simulink model "ID"  (R2024b)
settings: Solver=FixedStepDiscrete  StartTime=0.0  StopTime=Inf  FixedStep=0.001  RelTol=1e-3
model workspace (MAT data in the model file):
  robot : robotics.RigidBodyTree (value not decoded)
libraries: robotmaniplib x3
settings Model: Creator=sung  LastModifiedBy=sung
settings HardwareCC: ProdBitPerLong=64  ProdHWDeviceType=Intel->x86-64 (Linux 64)
settings RTWCC: GenCodeOnly=on  Toolchain=CMake

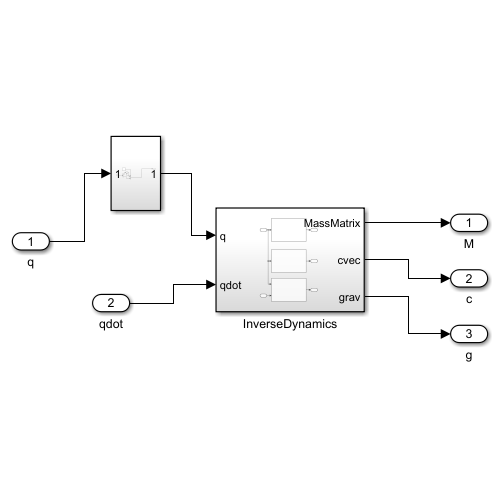
[thumbnail: Simulink's stored preview of the top-level diagram]
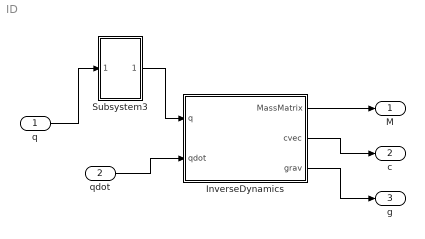
== system ID ==
  q : Inport
  qdot : Inport  Port=2
  InverseDynamics : Subsystem
  Subsystem3 : Subsystem
  M : Outport
  c : Outport  Port=2
  g : Outport  Port=3
  wires:
  q/1 -> Subsystem3/1(In1)
  qdot/1 -> InverseDynamics/2(qdot)
  InverseDynamics/1(MassMatrix) -> M/1
  InverseDynamics/2(cvec) -> c/1
  InverseDynamics/3(grav) -> g/1
  Subsystem3/1(Out1) -> InverseDynamics/1(q)

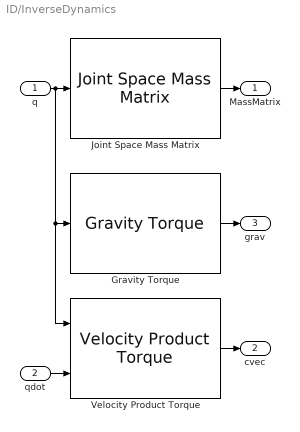
== system ID/InverseDynamics ==
  q : Inport
  qdot : Inport  Port=2
  Gravity Torque : robotmaniplib/Gravity Torque  RigidBodyTree=robot  SimulateUsing=Code generation
  Joint Space Mass Matrix : robotmaniplib/Joint Space Mass Matrix  RigidBodyTree=robot  SimulateUsing=Code generation
  Velocity Product Torque : robotmaniplib/Velocity Product Torque  RigidBodyTree=robot  SimulateUsing=Code generation
  MassMatrix : Outport
  cvec : Outport  Port=2
  grav : Outport  Port=3
  wires:
  Velocity Product Torque/1 -> cvec/1
  Joint Space Mass Matrix/1 -> MassMatrix/1
  Gravity Torque/1 -> grav/1
  q/1 -> Velocity Product Torque/1, Gravity Torque/1, Joint Space Mass Matrix/1
  qdot/1 -> Velocity Product Torque/2

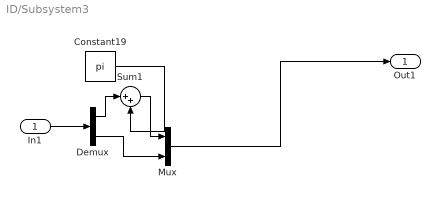
== system ID/Subsystem3 ==
  In1 : Inport
  Constant19 : Constant  Value=pi
  Demux : Demux  Outputs=[1,11]
  Mux : Mux  Inputs=[1,11]
  Sum1 : Sum  Inputs=|++
  Out1 : Outport
  wires:
  Constant19/1 -> Sum1/2
  Demux/2 -> Mux/2
  Mux/1 -> Out1/1
  In1/1 -> Demux/1
  Demux/1 -> Sum1/1
  Sum1/1 -> Mux/1
